simulink model "hw_1"  (R2014b)
settings: Solver=ode45  StartTime=0.0  StopTime=5  RelTol=1e-3
settings Model: Creator=treasersmac  LastModifiedBy=treasersmac

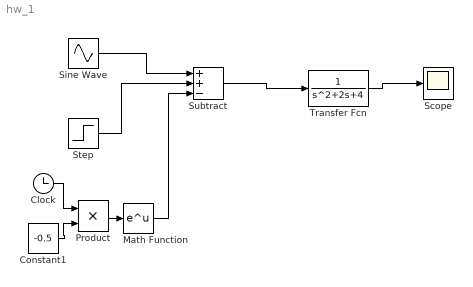
== system hw_1 ==
  Clock : Clock
  Constant1 : Constant  Value=-0.5
  Math Function : Math  SaturateOnIntegerOverflow=on
  Product : Product
  Scope : Scope
  Sine Wave : Sin  Amplitude=5  SampleTime=0
  Step : Step  SampleTime=0
  Subtract : Sum  Inputs=++-
  Transfer Fcn : TransferFcn  Numerator=[0 0 1]  Denominator=[1 2 4]
  wires:
  Transfer Fcn/1 -> Scope/1
  Step/1 -> Subtract/2
  Sine Wave/1 -> Subtract/1
  Math Function/1 -> Subtract/3
  Subtract/1 -> Transfer Fcn/1
  Clock/1 -> Product/1
  Constant1/1 -> Product/2
  Product/1 -> Math Function/1
